simulink model "Lead_Guidance_Method"  (R2024b)
settings: Solver=FixedStepAuto  StartTime=0.0  StopTime=200  FixedStep=0.01  RelTol=1e-3
settings Model: Creator=Acer  LastModifiedBy=Acer
settings DataIOCC: ReturnWorkspaceOutputs=off

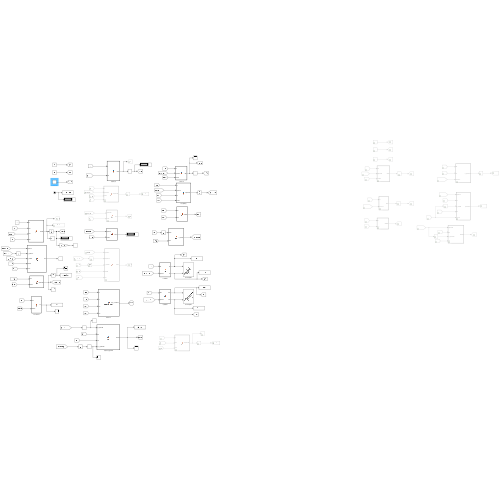
[thumbnail: Simulink's stored preview of the top-level diagram]
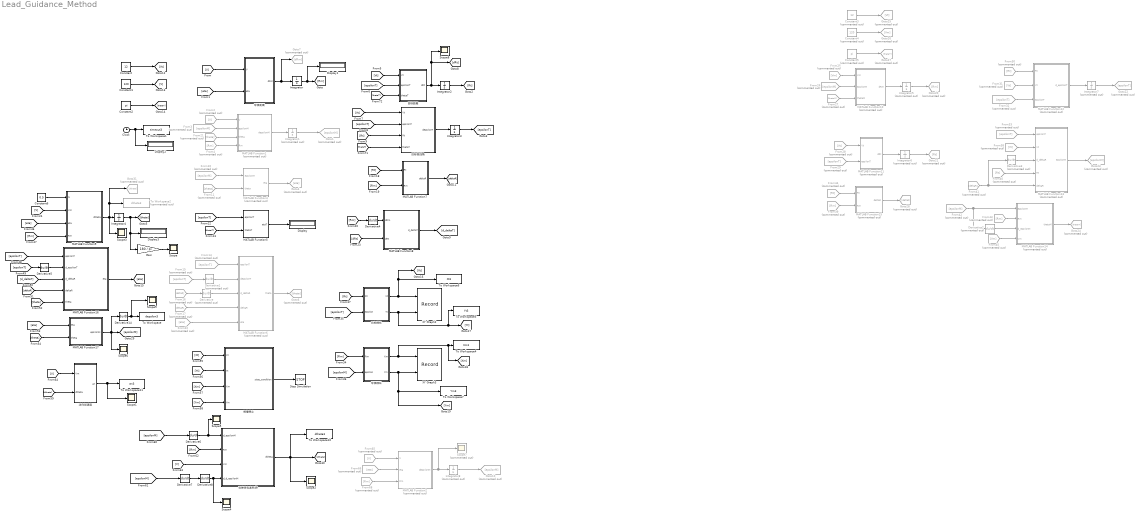
== system Lead_Guidance_Method ==
  Clock : Clock
  Constant : Constant  Value=12
  Constant1 : Constant  Value=120
  Constant2 : Constant  Value=pi
  Constant3 : Constant  Commented=on  Value=12
  Constant4 : Constant  Commented=on  Value=120
  Constant5 : Constant  Commented=on  Value=pi
  Constant6 : Constant  Value=0.5
  Derivative{,1..3} (4 alike) : Derivative  Commented=on
  Derivative{4..8,14} (6 alike) : Derivative
  Display{,1..3} (4 alike) : Display
  From{3,10,26,42} (4 alike) : From  Commented=on  GotoTag=epsilonM
  From11 : From  Commented=on  GotoTag=theta
  From{14..15,29,32..33} (5 alike) : From  Commented=on  GotoTag=epsilonT
  From16 : From  Commented=on  GotoTag=deltaR
  From17 : From  Commented=on  GotoTag=deltaR
  From2 : From  Commented=on  GotoTag=V
  From21 : From  Commented=on  GotoTag=theta
  From22 : From  Commented=on  GotoTag=eta
  From25 : From  Commented=on  GotoTag=Vm
  From27 : From  Commented=on  GotoTag=thetaM
  From28 : From  Commented=on  GotoTag=Vt
  From30 : From  Commented=on  GotoTag=Rt
  From31 : From  Commented=on  GotoTag=Vt
  From38 : From  Commented=on  GotoTag=Vt
  From{4,39,43,68} (4 alike) : From  Commented=on  GotoTag=Rm
  From40 : From  Commented=on  GotoTag=Rt
  From41 : From  Commented=on  GotoTag=deltaR
  From44 : From  Commented=on  GotoTag=Rt
  From45 : From  Commented=on  GotoTag=Vm
  From65 : From  Commented=on  GotoTag=V
  From66 : From  Commented=on  GotoTag=eta
  Gain : Gain  Gain=180 / pi
  Goto1 : Goto  Commented=on  GotoTag=epsilonM
  Goto10 : Goto  Commented=on  GotoTag=epsilonM
  Goto20 : Goto  Commented=on  GotoTag=Rm
  Goto21 : Goto  Commented=on  GotoTag=Rt
  Goto22 : Goto  Commented=on  GotoTag=epsilonT
  Goto23 : Goto  Commented=on  GotoTag=epsilonM
  Goto24 : Goto  Commented=on  GotoTag=thetaM
  Goto25 : Goto  Commented=on  GotoTag=Vt
  Goto26 : Goto  Commented=on  GotoTag=Vm
  Goto27 : Goto  Commented=on  GotoTag=thetaT
  Goto28 : Goto  Commented=on  GotoTag=deltaR
  Goto31 : Goto  Commented=on  GotoTag=dtheta
  Goto4 : Goto  Commented=on  GotoTag=eta
  Goto6 : Goto  Commented=on  GotoTag=theta
  Goto7 : Goto  Commented=on  GotoTag=dRm
  Integrator : Integrator  InitialCondition=50
  Integrator1 : Integrator  Commented=on  InitialCondition=65*pi/180
  Integrator2 : Integrator  InitialCondition=3000
  Integrator3 : Integrator  InitialCondition=70 * pi / 180
  Integrator4 : Integrator  InitialCondition=70 * pi /180
  Integrator5 : Integrator  Commented=on  InitialCondition=50
  Integrator6 : Integrator  Commented=on  InitialCondition=3000
  Integrator7 : Integrator  Commented=on  InitialCondition=60 * pi /180
  Integrator8 : Integrator  Commented=on  InitialCondition=65*pi/180
  MATLAB Function1 : MATLAB Function  Commented=on  TreatAsAtomicUnit=on
  MATLAB Function10 : MATLAB Function  Commented=on  TreatAsAtomicUnit=on
  MATLAB Function11 : MATLAB Function  Commented=on  TreatAsAtomicUnit=on
  MATLAB Function12 : MATLAB Function  Commented=on  TreatAsAtomicUnit=on
  MATLAB Function13 : MATLAB Function  Commented=on  TreatAsAtomicUnit=on
  MATLAB Function14 : MATLAB Function  Commented=on  TreatAsAtomicUnit=on
  MATLAB Function15 : MATLAB Function  Commented=on  TreatAsAtomicUnit=on
  MATLAB Function16 : MATLAB Function  TreatAsAtomicUnit=on
  MATLAB Function17 : MATLAB Function  TreatAsAtomicUnit=on
  MATLAB Function2 : MATLAB Function  Commented=on  TreatAsAtomicUnit=on
  MATLAB Function4 : MATLAB Function  Commented=on  TreatAsAtomicUnit=on
  MATLAB Function5 : MATLAB Function  TreatAsAtomicUnit=on
  MATLAB Function6 : MATLAB Function  Commented=on  TreatAsAtomicUnit=on
  MATLAB Function7 : MATLAB Function  TreatAsAtomicUnit=on
  MATLAB Function8 : MATLAB Function  TreatAsAtomicUnit=on
  MATLAB Function9 : MATLAB Function  TreatAsAtomicUnit=on
  Scope{,1..6,8..9} (9 alike) : Scope
  Scope7 : Scope  Commented=on
  Stop Simulation : Stop
  To Workspace : ToWorkspace  VariableName=depsilon3  SaveFormat=Timeseries  SampleTime=-1
  To Workspace1 : ToWorkspace  VariableName=timeout3  SaveFormat=Timeseries  SampleTime=-1
  To Workspace10 : ToWorkspace  VariableName=dtheta3  SaveFormat=Timeseries  SampleTime=-1
  To Workspace11 : ToWorkspace  VariableName=an3  SaveFormat=Timeseries  SampleTime=-1
  To Workspace2 : ToWorkspace  Commented=on  VariableName=dtheta3  SaveFormat=Timeseries  SampleTime=-1
  To Workspace4 : ToWorkspace  VariableName=Xm3  SaveFormat=Timeseries  SampleTime=-1
  To Workspace5 : ToWorkspace  VariableName=Yt3  SaveFormat=Timeseries  SampleTime=-1
  To Workspace6 : ToWorkspace  VariableName=Xt3  SaveFormat=Timeseries  SampleTime=-1
  To Workspace7 : ToWorkspace  VariableName=Ym3  SaveFormat=Timeseries  SampleTime=-1
  XY Graph2 : Record  FileSettingsInternal="{\"entries\":[{\"content\":{\"excelSettings\":{\"content\":{},\"type\":\"Streamout.ExcelSettings\"}},\"type\":\"Streamout.FileSettingStorage\",\"uuid\":\"\"}],\"packageUris\":[\"http:\\/\\/schema.mathworks.com\\/mf0\\/streamout_blocks\\/R2020a\"],\"version\":\"1.0\"}"  Layout=[1 1]  SignalsInternal="{\"entries\":[{\"content\":{\"signals\":[{\"content\":{\"blockPath\":[],\"dimensions\":[1],\"domain\":\"\",\"lineColor\":\"#b746ff\",\"lineWidth\":2,\"plots\":[ 1 ],\"port\":1,\"signalID\":1,\"signalName\":\"目标横纵:1\"},\"type\":\"RecordBlkView.Signal\",\"uuid\":\"\"},{\"content\":{\"blockPath\":[],\"dimensions\":[1],\"domain\":\"\",\"lineColor\":\"#64d413\",\"lineWidth\":2,\"plots\":[ 1 ],\"port\":2,\"signalID\":2,\"signalName\":\"目标横纵:2\"},\"type\":\"RecordBlkView.Signal\",\"uuid\":\"\"}]},\"type\":\"RecordBlkView.InputSignals\",\"uuid\":\"\"}],\"packageUris\":[\"http:\\/\\/schema.mathworks.com\\/mf0\\/streamout_blocks\\/R2020a\"],\"version\":\"1.0\"}"  VisualizationBindings="{\"xyplotplugin\":{\"info\":[{\"series\":[{\"bindingParametersList\":[{\"parameter\":\"X-Axis\",\"signalID\":1,\"signalName\":\"目标横纵:1\"},{\"parameter\":\"Y-Axis\",\"signalID\":2,\"signalName\":\"目标横纵:2\"}],\"seriesID\":0}],\"subplotID\":1}]}}"  CompatibilityTag=XY
  XY Graph3 : Record  FileSettingsInternal="{\"entries\":[{\"content\":{\"excelSettings\":{\"content\":{},\"type\":\"Streamout.ExcelSettings\"}},\"type\":\"Streamout.FileSettingStorage\",\"uuid\":\"\"}],\"packageUris\":[\"http:\\/\\/schema.mathworks.com\\/mf0\\/streamout_blocks\\/R2020a\"],\"version\":\"1.0\"}"  Layout=[1 1]  SignalsInternal="{\"entries\":[{\"content\":{\"signals\":[{\"content\":{\"blockPath\":[],\"dimensions\":[1],\"domain\":\"\",\"lineColor\":\"#ff13a6\",\"lineWidth\":2,\"plots\":[ 1 ],\"port\":1,\"signalID\":1,\"signalName\":\"导弹横纵:1\"},\"type\":\"RecordBlkView.Signal\",\"uuid\":\"\"},{\"content\":{\"blockPath\":[],\"dimensions\":[1],\"domain\":\"\",\"lineColor\":\"#fe330a\",\"lineWidth\":2,\"plots\":[ 1 ],\"port\":2,\"signalID\":2,\"signalName\":\"导弹横纵:2\"},\"type\":\"RecordBlkView.Signal\",\"uuid\":\"\"}]},\"type\":\"RecordBlkView.InputSignals\",\"uuid\":\"\"}],\"packageUris\":[\"http:\\/\\/schema.mathworks.com\\/mf0\\/streamout_blocks\\/R2020a\"],\"version\":\"1.0\"}"  VisualizationBindings="{\"xyplotplugin\":{\"info\":[{\"series\":[{\"bindingParametersList\":[{\"parameter\":\"X-Axis\",\"signalID\":1,\"signalName\":\"导弹横纵:1\"},{\"parameter\":\"Y-Axis\",\"signalID\":2,\"signalName\":\"导弹横纵:2\"}],\"seriesID\":0}],\"subplotID\":1}]}}"  CompatibilityTag=XY
  导弹横纵 : MATLAB Function  TreatAsAtomicUnit=on
  导弹距离 : MATLAB Function  TreatAsAtomicUnit=on
  导弹转弯速率dθ : MATLAB Function  TreatAsAtomicUnit=on
  法向加速度 : MATLAB Function  TreatAsAtomicUnit=on
  目标横纵 : MATLAB Function  TreatAsAtomicUnit=on
  目标视线角 : MATLAB Function  TreatAsAtomicUnit=on
  目标距离 : MATLAB Function  TreatAsAtomicUnit=on
  相撞停止 : MATLAB Function  TreatAsAtomicUnit=on
  wires:
  导弹距离/1(dRm) -> Goto7/1, Integrator/1
  [Rt] -> 目标视线角/3(Rt)
  [Vt] -> 目标视线角/1(Vt)
  From2/1 -> MATLAB Function1/1(V)
  From4/1 -> MATLAB Function1/4(Rm)
  MATLAB Function1/1(depsilonM) -> Integrator1/1
  Integrator1/1 -> Goto1/1
  Integrator/1 -> Display1/1, [Rm]
  [V] -> 导弹距离/1(V)
  [Vt] -> 目标距离/1(Vt)
  目标距离/1(dRt) -> Integrator2/1, Scope8/1, [dRt]
  Integrator2/1 -> [Rt]
  目标视线角/1(depsilonT) -> Integrator3/1
  Integrator3/1 -> [epsilonT]
  From11/1 -> MATLAB Function4/2(theta)
  [thetaT] -> MATLAB Function5/2(thetaT)
  [epsilonT] -> MATLAB Function5/1(epsilonT)
  MATLAB Function5/1(etaT) -> Display/1
  MATLAB Function7/1(deltaR) -> [deltaR]
  [Rm] -> MATLAB Function7/2(Rm)
  [Rt] -> MATLAB Function7/1(Rt)
  Constant/1 -> [Vt]
  Constant1/1 -> [V]
  Constant2/1 -> [thetaT]
  [epsilonM] -> 导弹横纵/2(epsilon)
  导弹横纵/1(Xm) -> [Xm], To Workspace4/1, XY Graph3/1
  [Rt] -> 目标横纵/1(Rt)
  [Rm] -> 导弹横纵/1(Rm)
  导弹横纵/2(Ym) -> [Ym], To Workspace7/1, XY Graph3/2
  目标横纵/2(Yt) -> To Workspace5/1, [Yt], XY Graph2/2
  目标横纵/1(Xt) -> XY Graph2/1, To Workspace6/1, [Xt]
  [epsilonT] -> 目标横纵/2(epsilon)
  Clock/1 -> Display2/1, To Workspace1/1
  MATLAB Function10/1(dRm) -> Integrator5/1
  Constant4/1 -> Goto26/1
  Constant5/1 -> Goto27/1
  Constant3/1 -> Goto25/1
  From43/1 -> MATLAB Function14/2(Rm)
  Derivative2/1 -> MATLAB Function14/3(d_epsilonM)
  From42/1 -> Derivative2/1, MATLAB Function14/1(epsilonM)
  From45/1 -> MATLAB Function14/4(Vm)
  MATLAB Function14/1(thetaM) -> Goto24/1
  From41/1 -> Derivative3/1, MATLAB Function13/5(deltaR)
  From40/1 -> MATLAB Function13/4(Rt)
  Integrator5/1 -> Goto20/1
  From25/1 -> MATLAB Function10/1(Vm)
  From26/1 -> MATLAB Function10/2(epsilonM)
  From27/1 -> MATLAB Function10/3(thetaM)
  MATLAB Function12/1(d_epsilonT) -> Integrator7/1
  Integrator7/1 -> Goto22/1
  From30/1 -> MATLAB Function12/1(Rt)
  From31/1 -> MATLAB Function12/2(Vt)
  From28/1 -> MATLAB Function11/1(Vt)
  From29/1 -> MATLAB Function11/2(epsilonT)
  MATLAB Function11/1(dRt) -> Integrator6/1
  Integrator6/1 -> Goto21/1
  From33/1 -> MATLAB Function13/1(epsilonT)
  From38/1 -> MATLAB Function13/2(Vt)
  Derivative3/1 -> MATLAB Function13/3(d_deltaR)
  MATLAB Function13/1(epsilonM) -> Goto23/1
  From32/1 -> MATLAB Function12/3(epsilonT)
  From44/1 -> MATLAB Function15/1(Rt)
  From39/1 -> MATLAB Function15/2(Rm)
  MATLAB Function15/1(deltaR) -> Goto28/1
  From14/1 -> MATLAB Function6/1(epsilonT)
  Derivative/1 -> MATLAB Function6/3(d_deltaR)
  From17/1 -> MATLAB Function6/4(deltaR)
  From22/1 -> MATLAB Function6/5(eta)
  MATLAB Function6/1(theta) -> Goto6/1
  From16/1 -> Derivative/1
  Derivative1/1 -> MATLAB Function6/2(depsilonT)
  From15/1 -> Derivative1/1
  From3/1 -> MATLAB Function1/2(epsilonM)
  From21/1 -> MATLAB Function1/3(theta)
  [epsilonT] -> 目标距离/2(epsilonT)
  [epsilonT] -> 目标视线角/2(epsilonT)
  [eta] -> 导弹距离/2(eta)
  MATLAB Function8/1(d_deltaT) -> [d_deltaT]
  Constant6/1 -> MATLAB Function9/1(N)
  [V] -> MATLAB Function9/2(Vm)
  [eta] -> MATLAB Function9/3(eta)
  [Rm] -> MATLAB Function9/4(Rm)
  MATLAB Function9/1(dtheta) -> To Workspace2/1, Goto31/1, Scope3/1, Integrator4/1
  Integrator4/1 -> Gain/1, Display3/1, [theta]
  [epsilonT] -> MATLAB Function16/1(epsilonT)
  [epsilonT] -> Derivative5/1
  [d_deltaT] -> MATLAB Function16/3(d_deltaR)
  [deltaR] -> MATLAB Function16/4(deltaR)
  [theta] -> MATLAB Function16/5(theta)
  MATLAB Function16/1(eta) -> [eta]
  [Rm] -> Derivative4/1
  Derivative4/1 -> MATLAB Function8/1(dRm)
  Derivative5/1 -> MATLAB Function16/2(d_epsilonT)
  [dRt] -> MATLAB Function8/2(dRt)
  From10/1 -> MATLAB Function4/1(epsilonM)
  MATLAB Function4/1(eta) -> Goto4/1
  [theta] -> MATLAB Function17/2(theta)
  [eta] -> MATLAB Function17/1(eta)
  MATLAB Function17/1(epsilonM) -> Scope6/1, [epsilonM], Derivative14/1
  相撞停止/1(stop_condition) -> Stop Simulation/1
  [Xm] -> 相撞停止/3(Xm)
  [Xt] -> 相撞停止/1(Xt)
  [Yt] -> 相撞停止/2(Yt)
  [Ym] -> 相撞停止/4(Ym)
  [V] -> 法向加速度/1(Vm)
  导弹转弯速率dθ/1(dtheta) -> To Workspace10/1, Scope2/1, [dtheta]
  [dtheta] -> 法向加速度/2(dtheta)
  法向加速度/1(an) -> Scope1/1, To Workspace11/1
  Gain/1 -> Scope/1
  Derivative14/1 -> Scope9/1, To Workspace/1
  [thetaT] -> 目标视线角/4(thetaT)
  [thetaT] -> 目标距离/3(thetaT)
  [epsilonM] -> Derivative6/1
  Derivative6/1 -> Scope5/1, 导弹转弯速率dθ/1(d_epsilonM)
  Derivative7/1 -> Derivative8/1
  Derivative8/1 -> Scope4/1, 导弹转弯速率dθ/4(d_d_epsilonM)
  [epsilonM] -> Derivative7/1
  [Rm] -> 导弹转弯速率dθ/2(Rm)
  [V] -> 导弹转弯速率dθ/3(Vm)
  MATLAB Function2/1(depsilonM) -> Scope7/1, Integrator8/1
  From68/1 -> MATLAB Function2/3(Rm)
  Integrator8/1 -> Goto10/1
  From65/1 -> MATLAB Function2/1(V)
  From66/1 -> MATLAB Function2/2(eta)

== matlab function Lead_Guidance_Method/MATLAB Function10 ==
  data: Vm input; dRm output; epsilonM input; thetaM input
function dRm = fcn(Vm, epsilonM, thetaM)

dRm = Vm * cos(epsilonM - thetaM);

== matlab function Lead_Guidance_Method/MATLAB Function11 ==
  data: Vt input; dRt output; epsilonT input
function dRt = fcn(Vt, epsilonT)

dRt = -(Vt * cos(epsilonT));

== matlab function Lead_Guidance_Method/MATLAB Function12 ==
  data: Rt input; d_epsilonT output; Vt input; epsilonT input
function d_epsilonT = fcn(Rt, Vt, epsilonT)

d_epsilonT = Vt * sin(epsilonT) / Rt;

== matlab function Lead_Guidance_Method/MATLAB Function13 ==
  data: epsilonT input; epsilonM output; Vt input; d_deltaR input; Rt input; deltaR input
function epsilonM = fcn(epsilonT, Vt, d_deltaR, Rt, deltaR)

epsilonM = epsilonT - ((Vt * sin(epsilonT) * deltaR) / (d_deltaR * Rt));

== matlab function Lead_Guidance_Method/目标横纵 ==
  data: Rt input; Xt output; epsilon input; Yt output
function [Xt, Yt] = fcn(Rt, epsilon)

Xt = Rt * cos(epsilon);
Yt = Rt * sin(epsilon);

== matlab function Lead_Guidance_Method/导弹横纵 ==
  data: Rm input; Xm output; epsilon input; Ym output
function [Xm, Ym] = fcn(Rm, epsilon)

Xm = Rm * cos(epsilon);
Ym = Rm * sin(epsilon);

== matlab function Lead_Guidance_Method/MATLAB Function1 ==
  data: V input; depsilonM output; epsilonM input; theta input; Rm input
function depsilonM = fcn(V, epsilonM, theta, Rm)

    depsilonM = -(V * sin(epsilonM - theta) / Rm);
end

== matlab function Lead_Guidance_Method/MATLAB Function14 ==
  data: epsilonM input; thetaM output; Rm input; d_epsilonM input; Vm input
function thetaM = fcn(epsilonM, Rm, d_epsilonM, Vm)

thetaM = epsilonM + asin(Rm * d_epsilonM / Vm);

== matlab function Lead_Guidance_Method/MATLAB Function15 ==
  data: Rt input; deltaR output; Rm input
function deltaR = fcn(Rt, Rm)

deltaR = Rt - Rm;

== matlab function Lead_Guidance_Method/MATLAB Function16 ==
  data: eta output; epsilonT input; d_epsilonT input; d_deltaR input; deltaR input; theta input
function eta = fcn(epsilonT, d_epsilonT, d_deltaR, deltaR, theta)

eta = epsilonT - (d_epsilonT * deltaR / d_deltaR) - theta;

== matlab function Lead_Guidance_Method/MATLAB Function17 ==
  data: eta input; epsilonM output; theta input
function epsilonM = fcn(eta, theta)

epsilonM = eta + theta;

== matlab function Lead_Guidance_Method/相撞停止 ==
  data: Xt input; stop_condition output; Yt input; Xm input; Ym input
function stop_condition = distance_check(Xt, Yt, Xm, Ym)
    
    distance = sqrt((Xt - Xm)^2 + (Yt - Ym)^2);
    stop_condition = distance < 1;
    
end

== matlab function Lead_Guidance_Method/导弹转弯速率dθ ==
  data: d_epsilonM input; Rm input; Vm input; d_d_epsilonM input; dtheta output
function dtheta = fcn(d_epsilonM, Rm, Vm, d_d_epsilonM)
    dtheta = 2 * d_epsilonM + Rm * d_d_epsilonM/ Vm;
end

== matlab function Lead_Guidance_Method/法向加速度 ==
  data: Vm input; an output; dtheta input
function an = fcn(Vm, dtheta)
    an = Vm * dtheta;
end

== matlab function Lead_Guidance_Method/MATLAB Function2 ==
  data: V input; depsilonM output; eta input; Rm input
function depsilonM = fcn(V, eta, Rm)

    depsilonM = -(V * sin(eta) / Rm);
end

== matlab function Lead_Guidance_Method/导弹距离 ==
  data: V input; dRm output; eta input
function dRm = fcn(V, eta)

    dRm = V * cos(eta);
end

== matlab function Lead_Guidance_Method/目标距离 ==
  data: Vt input; dRt output; epsilonT input; thetaT input
function dRt = fcn(Vt, epsilonT, thetaT)

    dRt = Vt * cos(epsilonT - thetaT);
end

== matlab function Lead_Guidance_Method/目标视线角 ==
  data: Vt input; depsilonT output; epsilonT input; Rt input; thetaT input
function depsilonT = fcn(Vt, epsilonT, Rt, thetaT)

    depsilonT = - ((Vt * sin(epsilonT - thetaT)) / Rt);
end

== matlab function Lead_Guidance_Method/MATLAB Function4 ==
  data: epsilonM input; eta output; theta input
function eta = fcn(epsilonM, theta)

eta = epsilonM - theta;

== matlab function Lead_Guidance_Method/MATLAB Function5 ==
  data: epsilonT input; etaT output; thetaT input
function etaT = fcn(epsilonT, thetaT)

etaT = epsilonT - thetaT;

== matlab function Lead_Guidance_Method/MATLAB Function6 ==
  data: epsilonT input; theta output; depsilonT input; d_deltaR input; deltaR input; eta input
function theta = fcn(epsilonT, depsilonT, d_deltaR, deltaR, eta)

theta = epsilonT - ((depsilonT / d_deltaR ) * deltaR) - eta;

== matlab function Lead_Guidance_Method/MATLAB Function7 ==
  data: Rt input; deltaR output; Rm input
function deltaR = fcn(Rt, Rm)

deltaR = Rt - Rm;

== matlab function Lead_Guidance_Method/MATLAB Function8 ==
  data: dRm input; d_deltaT output; dRt input
function d_deltaT = fcn(dRm, dRt)

d_deltaT = dRt - dRm;

== matlab function Lead_Guidance_Method/MATLAB Function9 ==
  data: N input; dtheta output; Vm input; eta input; Rm input
function dtheta = fcn(N, Vm, eta, Rm)

dtheta = (-N) * Vm * sin(eta) / Rm;
